simulink model "CMOS_Kernel_Memory_Sync"  (R2023b)
settings: Solver=VariableStepAuto  StartTime=0.0  StopTime=30000000  RelTol=1e-3
values from neighbouring files (symbols this model uses):
  AmountOfPixelsPerScanline = 400    [Kernel_Setup_Script.m]
  AmountOfRamBlocksScanlines = 5    [Kernel_Setup_Script.m]
  AmountOfRamBlocksScanlinesOffset = AmountOfRamBlocksScanlines - 1    (= 4)    [Kernel_Setup_Script.m]
  AmountOfScanlinePixels = 73700    [Kernel_Setup_Script.m]
  AmountOfScanlinePixelsOffset = AmountOfScanlinePixels - 1    (= 73699)    [Kernel_Setup_Script.m]
  AmountOfScanlines = 1100    [Kernel_Setup_Script.m]
  AmountOfScanlinesOffset = AmountOfScanlines - 1    (= 1099)    [Kernel_Setup_Script.m]
  AOPPK_Off = AmountOfPixelsPerScanline - 1    (= 399)    [Kernel_Setup_Script.m]
  AOPPS_Off = AmountOfPixelsPerScanline - 1    (= 399)    [Kernel_Setup_Script.m]
  FramePackOff_0 = FramePackOff_0 - ScanlineFifoCheck    [Kernel_Setup_Script.m]
  FramePackOff_1 = FramePackOff_1 - ScanlineFifoCheck    [Kernel_Setup_Script.m]
  FramePackOff_2 = FramePackOff_2 - ScanlineFifoCheck    [Kernel_Setup_Script.m]
  FramePackOff_3 = FramePackOff_3 - ScanlineFifoCheck    [Kernel_Setup_Script.m]
  FramePackOff_4 = FramePackOff_4 - ScanlineFifoCheck    [Kernel_Setup_Script.m]
  FramePackOff_5 = FramePackOff_5 - ScanlineFifoCheck    [Kernel_Setup_Script.m]
  KernelPackOff_0 = KernelPackOff_0 - KernelBitsPerRow    [Kernel_Setup_Script.m]
  KernelPackOff_1 = KernelPackOff_1 - KernelBitsPerRow    [Kernel_Setup_Script.m]
  KernelPackOff_2 = KernelPackOff_2 - KernelBitsPerRow    [Kernel_Setup_Script.m]
  KernelPackOff_3 = KernelPackOff_3 - KernelBitsPerRow    [Kernel_Setup_Script.m]
  Slice59DownTo48Top = (MsbOffset - (ScanlinePixelBitSizeController*1))    (= 59)    [Kernel_Setup_Script.m]
  Slice71DownTo60Top = (MsbOffset - (ScanlinePixelBitSizeController*0))    (= 71)    [Kernel_Setup_Script.m]
  TotalSectionsForFrames = AmountOfScanlines/AmountOfRamBlocksScanlines    (= 220)    [Kernel_Setup_Script.m]
  UltraRamRows = AmountOfPixelsPerScanline/ScanlineFifoCheck    [Kernel_Setup_Script.m]
  UltraRamRowsCeil = ceil(AmountOfPixelsPerScanline/ScanlineFifoCheck)    [Kernel_Setup_Script.m]
  UltraRamRowsKernel = AmountOfPixelsPerScanline/KernelBitsPerRow    (= 100)    [Kernel_Setup_Script.m]
  UltraRamRowsKernelCeil = ceil(AmountOfPixelsPerScanline/KernelBitsPerRow)    [Kernel_Setup_Script.m]
  UltraRamRowsMemorySectionOffset = UltraRamRowsCeil*AmountOfRamBlocksScanlines    [Kernel_Setup_Script.m]
  UltraRamRowsOffset = UltraRamRowsCeil - 1    [Kernel_Setup_Script.m]
undefined symbols (not defined in the file or in its folder): c, Down, sfvc784, Up, xck26
libraries: hdlBasic x4512, vmcUtilities x1
(part 8 of 39)

== system CMOS_Kernel_Memory_Sync/Memory Handler/Math/Kernel Result 3 ==
  Pixel Bus Input Offset 0 : Inport
  Pixel Bus Input Offset 1 : Inport  Port=2
  Pixel Bus Input Offset 2 : Inport  Port=3
  Pixel Bus Input Offset 3 : Inport  Port=4
  Pixel Bus Input Offset 4 : Inport  Port=5
  Weight Bus Input : Inport  Port=6
  Valid Bus Input : Inport  Port=7
  Hard Reset : Inport  Port=8
  Accumlator Kernel Results : Subsystem
  Accumulator Offset 0 : Subsystem
  Accumulator Offset 1 : Subsystem
  Accumulator Offset 2 : Subsystem
  Accumulator Offset 3 : Subsystem
  Accumulator Offset 4 : Subsystem
  Bus Selector : BusSelector  OutputSignals=signal1,signal2,signal3,signal4,signal5,signal6
  Delay Addition 1 : hdlBasic/Delay  rst=off  en=off  latency=1  reg_retiming=off  XmcBlockStatus=1  maskContainerNames=group1  block_type=delay  block_config=sysgen:Delay_config
  Delay Addition 2 : hdlBasic/Delay  rst=off  en=off  latency=1  reg_retiming=off  XmcBlockStatus=1  maskContainerNames=group1  block_type=delay  block_config=sysgen:Delay_config
  Delay Addition1 : hdlBasic/Delay  rst=off  en=off  latency=3  reg_retiming=off  XmcBlockStatus=1  maskContainerNames=group1  block_type=delay  block_config=sysgen:Delay_config
  Delay Addition{2..4,6..8} (6 alike) : hdlBasic/Delay  rst=off  en=off  latency=1  reg_retiming=off  XmcBlockStatus=1  maskContainerNames=group1  block_type=delay  block_config=sysgen:Delay_config
  Delay Addition5 : hdlBasic/Delay  rst=off  en=off  latency=3  reg_retiming=off  XmcBlockStatus=1  maskContainerNames=group1  block_type=delay  block_config=sysgen:Delay_config
  Multiple and Add Offset 0 : Subsystem
  Multiple and Add Offset 1 : Subsystem
  Multiple and Add Offset 2 : Subsystem
  Multiple and Add Offset 3 : Subsystem
  Multiple and Add Offset 4 : Subsystem
  Pixel Bus Offset {0..4} (5 alike) : BusSelector  OutputSignals=signal1,signal2,signal3,signal4,signal5,signal6,signal7,signal8,signal9,signal10,signal11,signal12
  Valid Selector : BusSelector  OutputSignals=signal1,signal2,signal3,signal4,signal5
  Weight Bus Offset {0..4} (5 alike) : BusSelector  OutputSignals=signal1,signal2,signal3,signal4,signal5,signal6,signal7,signal8,signal9,signal10,signal11,signal12
  Kernel Output : Outport
  Valid Kernel Output : Outport  Port=2
  wires:
  Multiple and Add Offset 4/1(Slice Out) -> Accumulator Offset 4/1(Input Value)
  Accumulator Offset 2/1(Accumulator Output) -> Accumlator Kernel Results/5(Slice Input 2)
  Accumulator Offset 0/2(Accumulator Valid) -> Accumlator Kernel Results/2(Slice Enable 0)
  Accumulator Offset 1/2(Accumulator Valid) -> Accumlator Kernel Results/4(Slice Enable 1)
  Multiple and Add Offset 2/2(Valid Out) -> Accumulator Offset 2/2(Input Valid)
  Accumulator Offset 0/1(Accumulator Output) -> Accumlator Kernel Results/1(Slice Input 0)
  Multiple and Add Offset 0/1(Slice Out) -> Accumulator Offset 0/1(Input Value)
  Multiple and Add Offset 1/1(Slice Out) -> Accumulator Offset 1/1(Input Value)
  Multiple and Add Offset 1/2(Valid Out) -> Accumulator Offset 1/2(Input Valid)
  Accumulator Offset 3/2(Accumulator Valid) -> Accumlator Kernel Results/8(Slice Enable 3)
  Multiple and Add Offset 0/2(Valid Out) -> Accumulator Offset 0/2(Input Valid)
  Multiple and Add Offset 4/2(Valid Out) -> Accumulator Offset 4/2(Input Valid)
  Accumulator Offset 3/1(Accumulator Output) -> Accumlator Kernel Results/7(Slice Input 3)
  Accumulator Offset 2/2(Accumulator Valid) -> Accumlator Kernel Results/6(Slice Enable 2)
  Multiple and Add Offset 3/2(Valid Out) -> Accumulator Offset 3/2(Input Valid)
  Accumulator Offset 4/1(Accumulator Output) -> Accumlator Kernel Results/9(Slice Input 4)
  Multiple and Add Offset 3/1(Slice Out) -> Accumulator Offset 3/1(Input Value)
  Multiple and Add Offset 2/1(Slice Out) -> Accumulator Offset 2/1(Input Value)
  Accumulator Offset 1/1(Accumulator Output) -> Accumlator Kernel Results/3(Slice Input 1)
  Accumulator Offset 4/2(Accumulator Valid) -> Accumlator Kernel Results/10(Slice Enable 4)
  Accumlator Kernel Results/2(Valid Kernel Output) -> Valid Kernel Output/1
  Accumlator Kernel Results/1(Kernel Output) -> Kernel Output/1
  Pixel Bus Input Offset 0/1 -> Pixel Bus Offset 0/1
  Pixel Bus Offset 0/1 -> Multiple and Add Offset 0/1(Pixel 0)  "<signal1>"
  Pixel Bus Offset 0/2 -> Multiple and Add Offset 0/3(Pixel 1)  "<signal2>"
  Pixel Bus Offset 0/3 -> Multiple and Add Offset 0/5(Pixel 2)  "<signal3>"
  Pixel Bus Offset 0/4 -> Multiple and Add Offset 0/7(Pixel 3)  "<signal4>"
  Pixel Bus Offset 0/5 -> Multiple and Add Offset 0/9(Pixel 4)  "<signal5>"
  Pixel Bus Offset 0/6 -> Multiple and Add Offset 0/11(Pixel 5)  "<signal6>"
  Pixel Bus Offset 0/7 -> Multiple and Add Offset 0/13(Pixel 6)  "<signal7>"
  Pixel Bus Offset 0/8 -> Multiple and Add Offset 0/15(Pixel 7)  "<signal8>"
  Pixel Bus Offset 0/9 -> Multiple and Add Offset 0/17(Pixel 8)  "<signal9>"
  Pixel Bus Offset 0/10 -> Multiple and Add Offset 0/19(Pixel 9)  "<signal10>"
  Pixel Bus Offset 0/11 -> Multiple and Add Offset 0/21(Pixel 10)  "<signal11>"
  Pixel Bus Offset 0/12 -> Multiple and Add Offset 0/23(Pixel 11)  "<signal12>"
  Weight Bus Offset 0/1 -> Multiple and Add Offset 0/2(Weight 0)  "<signal1>"
  Weight Bus Offset 0/2 -> Multiple and Add Offset 0/4(Weight 1)  "<signal2>"
  Weight Bus Offset 0/3 -> Multiple and Add Offset 0/6(Weight 2)  "<signal3>"
  Weight Bus Offset 0/4 -> Multiple and Add Offset 0/8(Weight 3)  "<signal4>"
  Weight Bus Offset 0/5 -> Multiple and Add Offset 0/10(Weight 4)  "<signal5>"
  Weight Bus Offset 0/6 -> Multiple and Add Offset 0/12(Weight 5)  "<signal6>"
  Weight Bus Offset 0/7 -> Multiple and Add Offset 0/14(Weight 6)  "<signal7>"
  Weight Bus Offset 0/8 -> Multiple and Add Offset 0/16(Weight 7)  "<signal8>"
  Weight Bus Offset 0/9 -> Multiple and Add Offset 0/18(Weight 8)  "<signal9>"
  Weight Bus Offset 0/10 -> Multiple and Add Offset 0/20(Weight 9)  "<signal10>"
  Weight Bus Offset 0/11 -> Multiple and Add Offset 0/22(Weight 10)  "<signal11>"
  Weight Bus Offset 0/12 -> Multiple and Add Offset 0/24(Weight 11)  "<signal12>"
  Weight Bus Offset 1/5 -> Multiple and Add Offset 1/10(Weight 4)  "<signal5>"
  Pixel Bus Offset 1/7 -> Multiple and Add Offset 1/13(Pixel 6)  "<signal7>"
  Pixel Bus Offset 1/6 -> Multiple and Add Offset 1/11(Pixel 5)  "<signal6>"
  Pixel Bus Offset 1/5 -> Multiple and Add Offset 1/9(Pixel 4)  "<signal5>"
  Pixel Bus Offset 1/3 -> Multiple and Add Offset 1/5(Pixel 2)  "<signal3>"
  Pixel Bus Offset 1/11 -> Multiple and Add Offset 1/21(Pixel 10)  "<signal11>"
  Weight Bus Offset 1/6 -> Multiple and Add Offset 1/12(Weight 5)  "<signal6>"
  Pixel Bus Offset 1/2 -> Multiple and Add Offset 1/3(Pixel 1)  "<signal2>"
  Weight Bus Offset 1/12 -> Multiple and Add Offset 1/24(Weight 11)  "<signal12>"
  Weight Bus Offset 1/1 -> Multiple and Add Offset 1/2(Weight 0)  "<signal1>"
  Pixel Bus Input Offset 1/1 -> Pixel Bus Offset 1/1
  Pixel Bus Offset 1/4 -> Multiple and Add Offset 1/7(Pixel 3)  "<signal4>"
  Weight Bus Offset 1/9 -> Multiple and Add Offset 1/18(Weight 8)  "<signal9>"
  Weight Bus Offset 1/10 -> Multiple and Add Offset 1/20(Weight 9)  "<signal10>"
  Weight Bus Offset 1/11 -> Multiple and Add Offset 1/22(Weight 10)  "<signal11>"
  Weight Bus Offset 1/4 -> Multiple and Add Offset 1/8(Weight 3)  "<signal4>"
  Pixel Bus Offset 1/1 -> Multiple and Add Offset 1/1(Pixel 0)  "<signal1>"
  Weight Bus Offset 1/8 -> Multiple and Add Offset 1/16(Weight 7)  "<signal8>"
  Weight Bus Offset 1/3 -> Multiple and Add Offset 1/6(Weight 2)  "<signal3>"
  Pixel Bus Offset 1/10 -> Multiple and Add Offset 1/19(Pixel 9)  "<signal10>"
  Pixel Bus Offset 1/8 -> Multiple and Add Offset 1/15(Pixel 7)  "<signal8>"
  Pixel Bus Offset 1/12 -> Multiple and Add Offset 1/23(Pixel 11)  "<signal12>"
  Weight Bus Offset 1/7 -> Multiple and Add Offset 1/14(Weight 6)  "<signal7>"
  Weight Bus Offset 1/2 -> Multiple and Add Offset 1/4(Weight 1)  "<signal2>"
  Pixel Bus Offset 1/9 -> Multiple and Add Offset 1/17(Pixel 8)  "<signal9>"
  Weight Bus Offset 2/5 -> Multiple and Add Offset 2/10(Weight 4)  "<signal5>"
  Pixel Bus Offset 2/7 -> Multiple and Add Offset 2/13(Pixel 6)  "<signal7>"
  Pixel Bus Offset 2/6 -> Multiple and Add Offset 2/11(Pixel 5)  "<signal6>"
  Pixel Bus Offset 2/5 -> Multiple and Add Offset 2/9(Pixel 4)  "<signal5>"
  Pixel Bus Offset 2/3 -> Multiple and Add Offset 2/5(Pixel 2)  "<signal3>"
  Pixel Bus Offset 2/11 -> Multiple and Add Offset 2/21(Pixel 10)  "<signal11>"
  Weight Bus Offset 2/6 -> Multiple and Add Offset 2/12(Weight 5)  "<signal6>"
  Pixel Bus Offset 2/2 -> Multiple and Add Offset 2/3(Pixel 1)  "<signal2>"
  Weight Bus Offset 2/12 -> Multiple and Add Offset 2/24(Weight 11)  "<signal12>"
  Weight Bus Offset 2/1 -> Multiple and Add Offset 2/2(Weight 0)  "<signal1>"
  Pixel Bus Input Offset 2/1 -> Pixel Bus Offset 2/1
  Pixel Bus Offset 2/4 -> Multiple and Add Offset 2/7(Pixel 3)  "<signal4>"
  Weight Bus Offset 2/9 -> Multiple and Add Offset 2/18(Weight 8)  "<signal9>"
  Weight Bus Offset 2/10 -> Multiple and Add Offset 2/20(Weight 9)  "<signal10>"
  Weight Bus Offset 2/11 -> Multiple and Add Offset 2/22(Weight 10)  "<signal11>"
  Weight Bus Offset 2/4 -> Multiple and Add Offset 2/8(Weight 3)  "<signal4>"
  Pixel Bus Offset 2/1 -> Multiple and Add Offset 2/1(Pixel 0)  "<signal1>"
  Weight Bus Offset 2/8 -> Multiple and Add Offset 2/16(Weight 7)  "<signal8>"
  Weight Bus Offset 2/3 -> Multiple and Add Offset 2/6(Weight 2)  "<signal3>"
  Pixel Bus Offset 2/10 -> Multiple and Add Offset 2/19(Pixel 9)  "<signal10>"
  Pixel Bus Offset 2/8 -> Multiple and Add Offset 2/15(Pixel 7)  "<signal8>"
  Pixel Bus Offset 2/12 -> Multiple and Add Offset 2/23(Pixel 11)  "<signal12>"
  Weight Bus Offset 2/7 -> Multiple and Add Offset 2/14(Weight 6)  "<signal7>"
  Weight Bus Offset 2/2 -> Multiple and Add Offset 2/4(Weight 1)  "<signal2>"
  Pixel Bus Offset 2/9 -> Multiple and Add Offset 2/17(Pixel 8)  "<signal9>"
  Weight Bus Offset 3/5 -> Multiple and Add Offset 3/10(Weight 4)  "<signal5>"
  Pixel Bus Offset 3/7 -> Multiple and Add Offset 3/13(Pixel 6)  "<signal7>"
  Pixel Bus Offset 3/6 -> Multiple and Add Offset 3/11(Pixel 5)  "<signal6>"
  Pixel Bus Offset 3/5 -> Multiple and Add Offset 3/9(Pixel 4)  "<signal5>"
  Pixel Bus Offset 3/3 -> Multiple and Add Offset 3/5(Pixel 2)  "<signal3>"
  Pixel Bus Offset 3/11 -> Multiple and Add Offset 3/21(Pixel 10)  "<signal11>"
  Weight Bus Offset 3/6 -> Multiple and Add Offset 3/12(Weight 5)  "<signal6>"
  Pixel Bus Offset 3/2 -> Multiple and Add Offset 3/3(Pixel 1)  "<signal2>"
  Weight Bus Offset 3/12 -> Multiple and Add Offset 3/24(Weight 11)  "<signal12>"
  Weight Bus Offset 3/1 -> Multiple and Add Offset 3/2(Weight 0)  "<signal1>"
  Pixel Bus Input Offset 3/1 -> Pixel Bus Offset 3/1
  Pixel Bus Offset 3/4 -> Multiple and Add Offset 3/7(Pixel 3)  "<signal4>"
  Weight Bus Offset 3/9 -> Multiple and Add Offset 3/18(Weight 8)  "<signal9>"
  Weight Bus Offset 3/10 -> Multiple and Add Offset 3/20(Weight 9)  "<signal10>"
  Weight Bus Offset 3/11 -> Multiple and Add Offset 3/22(Weight 10)  "<signal11>"
  Weight Bus Offset 3/4 -> Multiple and Add Offset 3/8(Weight 3)  "<signal4>"
  Pixel Bus Offset 3/1 -> Multiple and Add Offset 3/1(Pixel 0)  "<signal1>"
  Weight Bus Offset 3/8 -> Multiple and Add Offset 3/16(Weight 7)  "<signal8>"
  Weight Bus Offset 3/3 -> Multiple and Add Offset 3/6(Weight 2)  "<signal3>"
  Pixel Bus Offset 3/10 -> Multiple and Add Offset 3/19(Pixel 9)  "<signal10>"
  Pixel Bus Offset 3/8 -> Multiple and Add Offset 3/15(Pixel 7)  "<signal8>"
  Pixel Bus Offset 3/12 -> Multiple and Add Offset 3/23(Pixel 11)  "<signal12>"
  Weight Bus Offset 3/7 -> Multiple and Add Offset 3/14(Weight 6)  "<signal7>"
  Weight Bus Offset 3/2 -> Multiple and Add Offset 3/4(Weight 1)  "<signal2>"
  Pixel Bus Offset 3/9 -> Multiple and Add Offset 3/17(Pixel 8)  "<signal9>"
  Weight Bus Offset 4/5 -> Multiple and Add Offset 4/10(Weight 4)  "<signal5>"
  Pixel Bus Offset 4/7 -> Multiple and Add Offset 4/13(Pixel 6)  "<signal7>"
  Pixel Bus Offset 4/6 -> Multiple and Add Offset 4/11(Pixel 5)  "<signal6>"
  Pixel Bus Offset 4/5 -> Multiple and Add Offset 4/9(Pixel 4)  "<signal5>"
  Pixel Bus Offset 4/3 -> Multiple and Add Offset 4/5(Pixel 2)  "<signal3>"
  Pixel Bus Offset 4/11 -> Multiple and Add Offset 4/21(Pixel 10)  "<signal11>"
  Weight Bus Offset 4/6 -> Multiple and Add Offset 4/12(Weight 5)  "<signal6>"
  Pixel Bus Offset 4/2 -> Multiple and Add Offset 4/3(Pixel 1)  "<signal2>"
  Weight Bus Offset 4/12 -> Multiple and Add Offset 4/24(Weight 11)  "<signal12>"
  Weight Bus Offset 4/1 -> Multiple and Add Offset 4/2(Weight 0)  "<signal1>"
  Pixel Bus Input Offset 4/1 -> Pixel Bus Offset 4/1
  Pixel Bus Offset 4/4 -> Multiple and Add Offset 4/7(Pixel 3)  "<signal4>"
  Weight Bus Offset 4/9 -> Multiple and Add Offset 4/18(Weight 8)  "<signal9>"
  Weight Bus Offset 4/10 -> Multiple and Add Offset 4/20(Weight 9)  "<signal10>"
  Weight Bus Offset 4/11 -> Multiple and Add Offset 4/22(Weight 10)  "<signal11>"
  Weight Bus Offset 4/4 -> Multiple and Add Offset 4/8(Weight 3)  "<signal4>"
  Pixel Bus Offset 4/1 -> Multiple and Add Offset 4/1(Pixel 0)  "<signal1>"
  Weight Bus Offset 4/8 -> Multiple and Add Offset 4/16(Weight 7)  "<signal8>"
  Weight Bus Offset 4/3 -> Multiple and Add Offset 4/6(Weight 2)  "<signal3>"
  Pixel Bus Offset 4/10 -> Multiple and Add Offset 4/19(Pixel 9)  "<signal10>"
  Pixel Bus Offset 4/8 -> Multiple and Add Offset 4/15(Pixel 7)  "<signal8>"
  Pixel Bus Offset 4/12 -> Multiple and Add Offset 4/23(Pixel 11)  "<signal12>"
  Weight Bus Offset 4/7 -> Multiple and Add Offset 4/14(Weight 6)  "<signal7>"
  Weight Bus Offset 4/2 -> Multiple and Add Offset 4/4(Weight 1)  "<signal2>"
  Pixel Bus Offset 4/9 -> Multiple and Add Offset 4/17(Pixel 8)  "<signal9>"
  Valid Bus Input/1 -> Valid Selector/1
  Valid Selector/1 -> Multiple and Add Offset 0/25(Valid Data)  "<signal1>"
  Valid Selector/2 -> Multiple and Add Offset 1/25(Valid Data)  "<signal2>"
  Valid Selector/3 -> Multiple and Add Offset 2/25(Valid Data)  "<signal3>"
  Valid Selector/4 -> Multiple and Add Offset 3/25(Valid Data)  "<signal4>"
  Valid Selector/5 -> Multiple and Add Offset 4/25(Valid Data)  "<signal5>"
  Weight Bus Input/1 -> Bus Selector/1
  Bus Selector/5 -> Weight Bus Offset 4/1  "<signal5>"
  Bus Selector/4 -> Weight Bus Offset 3/1  "<signal4>"
  Bus Selector/3 -> Weight Bus Offset 2/1  "<signal3>"
  Bus Selector/2 -> Weight Bus Offset 1/1  "<signal2>"
  Bus Selector/1 -> Weight Bus Offset 0/1  "<signal1>"
  Delay Addition4/1 -> Accumulator Offset 4/3(Last Row), Accumulator Offset 3/3(Last Row), Accumulator Offset 2/3(Last Row), Accumulator Offset 1/3(Last Row), Accumulator Offset 0/3(Last Row)
  Delay Addition 2/1 -> Delay Addition2/1
  Delay Addition1/1 -> Delay Addition 2/1
  Delay Addition2/1 -> Delay Addition3/1
  Delay Addition3/1 -> Delay Addition4/1
  Bus Selector/6 -> Delay Addition1/1  "<signal6>"
  Delay Addition7/1 -> Delay Addition8/1
  Delay Addition 1/1 -> Delay Addition6/1
  Delay Addition5/1 -> Delay Addition 1/1
  Delay Addition6/1 -> Delay Addition7/1
  Delay Addition8/1 -> Accumlator Kernel Results/11(Reset Collector), Accumulator Offset 0/4(Hard Reset), Accumulator Offset 1/4(Hard Reset), Accumulator Offset 2/4(Hard Reset), Accumulator Offset 3/4(Hard Reset), Accumulator Offset 4/4(Hard Reset)
  Hard Reset/1 -> Delay Addition5/1

== system CMOS_Kernel_Memory_Sync/Memory Handler/Math/Kernel Result 4 ==
  Pixel Bus Input Offset 0 : Inport
  Pixel Bus Input Offset 1 : Inport  Port=2
  Pixel Bus Input Offset 2 : Inport  Port=3
  Pixel Bus Input Offset 3 : Inport  Port=4
  Pixel Bus Input Offset 4 : Inport  Port=5
  Weight Bus Input : Inport  Port=6
  Valid Bus Input : Inport  Port=7
  Hard Reset : Inport  Port=8
  Accumlator Kernel Results : Subsystem
  Accumulator Offset 0 : Subsystem
  Accumulator Offset 1 : Subsystem
  Accumulator Offset 2 : Subsystem
  Accumulator Offset 3 : Subsystem
  Accumulator Offset 4 : Subsystem
  Bus Selector : BusSelector  OutputSignals=signal1,signal2,signal3,signal4,signal5,signal6
  Delay Addition 1 : hdlBasic/Delay  rst=off  en=off  latency=1  reg_retiming=off  XmcBlockStatus=1  maskContainerNames=group1  block_type=delay  block_config=sysgen:Delay_config
  Delay Addition 2 : hdlBasic/Delay  rst=off  en=off  latency=1  reg_retiming=off  XmcBlockStatus=1  maskContainerNames=group1  block_type=delay  block_config=sysgen:Delay_config
  Delay Addition1 : hdlBasic/Delay  rst=off  en=off  latency=3  reg_retiming=off  XmcBlockStatus=1  maskContainerNames=group1  block_type=delay  block_config=sysgen:Delay_config
  Delay Addition{2..4,6..8} (6 alike) : hdlBasic/Delay  rst=off  en=off  latency=1  reg_retiming=off  XmcBlockStatus=1  maskContainerNames=group1  block_type=delay  block_config=sysgen:Delay_config
  Delay Addition5 : hdlBasic/Delay  rst=off  en=off  latency=3  reg_retiming=off  XmcBlockStatus=1  maskContainerNames=group1  block_type=delay  block_config=sysgen:Delay_config
  Multiple and Add Offset 0 : Subsystem
  Multiple and Add Offset 1 : Subsystem
  Multiple and Add Offset 2 : Subsystem
  Multiple and Add Offset 3 : Subsystem
  Multiple and Add Offset 4 : Subsystem
  Pixel Bus Offset {0..4} (5 alike) : BusSelector  OutputSignals=signal1,signal2,signal3,signal4,signal5,signal6,signal7,signal8,signal9,signal10,signal11,signal12
  Valid Selector : BusSelector  OutputSignals=signal1,signal2,signal3,signal4,signal5
  Weight Bus Offset {0..4} (5 alike) : BusSelector  OutputSignals=signal1,signal2,signal3,signal4,signal5,signal6,signal7,signal8,signal9,signal10,signal11,signal12
  Kernel Output : Outport
  Valid Kernel Output : Outport  Port=2
  wires:
  Multiple and Add Offset 4/1(Slice Out) -> Accumulator Offset 4/1(Input Value)
  Accumulator Offset 2/1(Accumulator Output) -> Accumlator Kernel Results/5(Slice Input 2)
  Accumulator Offset 0/2(Accumulator Valid) -> Accumlator Kernel Results/2(Slice Enable 0)
  Accumulator Offset 1/2(Accumulator Valid) -> Accumlator Kernel Results/4(Slice Enable 1)
  Multiple and Add Offset 2/2(Valid Out) -> Accumulator Offset 2/2(Input Valid)
  Accumulator Offset 0/1(Accumulator Output) -> Accumlator Kernel Results/1(Slice Input 0)
  Multiple and Add Offset 0/1(Slice Out) -> Accumulator Offset 0/1(Input Value)
  Multiple and Add Offset 1/1(Slice Out) -> Accumulator Offset 1/1(Input Value)
  Multiple and Add Offset 1/2(Valid Out) -> Accumulator Offset 1/2(Input Valid)
  Accumulator Offset 3/2(Accumulator Valid) -> Accumlator Kernel Results/8(Slice Enable 3)
  Multiple and Add Offset 0/2(Valid Out) -> Accumulator Offset 0/2(Input Valid)
  Multiple and Add Offset 4/2(Valid Out) -> Accumulator Offset 4/2(Input Valid)
  Accumulator Offset 3/1(Accumulator Output) -> Accumlator Kernel Results/7(Slice Input 3)
  Accumulator Offset 2/2(Accumulator Valid) -> Accumlator Kernel Results/6(Slice Enable 2)
  Multiple and Add Offset 3/2(Valid Out) -> Accumulator Offset 3/2(Input Valid)
  Accumulator Offset 4/1(Accumulator Output) -> Accumlator Kernel Results/9(Slice Input 4)
  Multiple and Add Offset 3/1(Slice Out) -> Accumulator Offset 3/1(Input Value)
  Multiple and Add Offset 2/1(Slice Out) -> Accumulator Offset 2/1(Input Value)
  Accumulator Offset 1/1(Accumulator Output) -> Accumlator Kernel Results/3(Slice Input 1)
  Accumulator Offset 4/2(Accumulator Valid) -> Accumlator Kernel Results/10(Slice Enable 4)
  Accumlator Kernel Results/2(Valid Kernel Output) -> Valid Kernel Output/1
  Accumlator Kernel Results/1(Kernel Output) -> Kernel Output/1
  Pixel Bus Input Offset 0/1 -> Pixel Bus Offset 0/1
  Pixel Bus Offset 0/1 -> Multiple and Add Offset 0/1(Pixel 0)  "<signal1>"
  Pixel Bus Offset 0/2 -> Multiple and Add Offset 0/3(Pixel 1)  "<signal2>"
  Pixel Bus Offset 0/3 -> Multiple and Add Offset 0/5(Pixel 2)  "<signal3>"
  Pixel Bus Offset 0/4 -> Multiple and Add Offset 0/7(Pixel 3)  "<signal4>"
  Pixel Bus Offset 0/5 -> Multiple and Add Offset 0/9(Pixel 4)  "<signal5>"
  Pixel Bus Offset 0/6 -> Multiple and Add Offset 0/11(Pixel 5)  "<signal6>"
  Pixel Bus Offset 0/7 -> Multiple and Add Offset 0/13(Pixel 6)  "<signal7>"
  Pixel Bus Offset 0/8 -> Multiple and Add Offset 0/15(Pixel 7)  "<signal8>"
  Pixel Bus Offset 0/9 -> Multiple and Add Offset 0/17(Pixel 8)  "<signal9>"
  Pixel Bus Offset 0/10 -> Multiple and Add Offset 0/19(Pixel 9)  "<signal10>"
  Pixel Bus Offset 0/11 -> Multiple and Add Offset 0/21(Pixel 10)  "<signal11>"
  Pixel Bus Offset 0/12 -> Multiple and Add Offset 0/23(Pixel 11)  "<signal12>"
  Weight Bus Offset 0/1 -> Multiple and Add Offset 0/2(Weight 0)  "<signal1>"
  Weight Bus Offset 0/2 -> Multiple and Add Offset 0/4(Weight 1)  "<signal2>"
  Weight Bus Offset 0/3 -> Multiple and Add Offset 0/6(Weight 2)  "<signal3>"
  Weight Bus Offset 0/4 -> Multiple and Add Offset 0/8(Weight 3)  "<signal4>"
  Weight Bus Offset 0/5 -> Multiple and Add Offset 0/10(Weight 4)  "<signal5>"
  Weight Bus Offset 0/6 -> Multiple and Add Offset 0/12(Weight 5)  "<signal6>"
  Weight Bus Offset 0/7 -> Multiple and Add Offset 0/14(Weight 6)  "<signal7>"
  Weight Bus Offset 0/8 -> Multiple and Add Offset 0/16(Weight 7)  "<signal8>"
  Weight Bus Offset 0/9 -> Multiple and Add Offset 0/18(Weight 8)  "<signal9>"
  Weight Bus Offset 0/10 -> Multiple and Add Offset 0/20(Weight 9)  "<signal10>"
  Weight Bus Offset 0/11 -> Multiple and Add Offset 0/22(Weight 10)  "<signal11>"
  Weight Bus Offset 0/12 -> Multiple and Add Offset 0/24(Weight 11)  "<signal12>"
  Weight Bus Offset 1/5 -> Multiple and Add Offset 1/10(Weight 4)  "<signal5>"
  Pixel Bus Offset 1/7 -> Multiple and Add Offset 1/13(Pixel 6)  "<signal7>"
  Pixel Bus Offset 1/6 -> Multiple and Add Offset 1/11(Pixel 5)  "<signal6>"
  Pixel Bus Offset 1/5 -> Multiple and Add Offset 1/9(Pixel 4)  "<signal5>"
  Pixel Bus Offset 1/3 -> Multiple and Add Offset 1/5(Pixel 2)  "<signal3>"
  Pixel Bus Offset 1/11 -> Multiple and Add Offset 1/21(Pixel 10)  "<signal11>"
  Weight Bus Offset 1/6 -> Multiple and Add Offset 1/12(Weight 5)  "<signal6>"
  Pixel Bus Offset 1/2 -> Multiple and Add Offset 1/3(Pixel 1)  "<signal2>"
  Weight Bus Offset 1/12 -> Multiple and Add Offset 1/24(Weight 11)  "<signal12>"
  Weight Bus Offset 1/1 -> Multiple and Add Offset 1/2(Weight 0)  "<signal1>"
  Pixel Bus Input Offset 1/1 -> Pixel Bus Offset 1/1
  Pixel Bus Offset 1/4 -> Multiple and Add Offset 1/7(Pixel 3)  "<signal4>"
  Weight Bus Offset 1/9 -> Multiple and Add Offset 1/18(Weight 8)  "<signal9>"
  Weight Bus Offset 1/10 -> Multiple and Add Offset 1/20(Weight 9)  "<signal10>"
  Weight Bus Offset 1/11 -> Multiple and Add Offset 1/22(Weight 10)  "<signal11>"
  Weight Bus Offset 1/4 -> Multiple and Add Offset 1/8(Weight 3)  "<signal4>"
  Pixel Bus Offset 1/1 -> Multiple and Add Offset 1/1(Pixel 0)  "<signal1>"
  Weight Bus Offset 1/8 -> Multiple and Add Offset 1/16(Weight 7)  "<signal8>"
  Weight Bus Offset 1/3 -> Multiple and Add Offset 1/6(Weight 2)  "<signal3>"
  Pixel Bus Offset 1/10 -> Multiple and Add Offset 1/19(Pixel 9)  "<signal10>"
  Pixel Bus Offset 1/8 -> Multiple and Add Offset 1/15(Pixel 7)  "<signal8>"
  Pixel Bus Offset 1/12 -> Multiple and Add Offset 1/23(Pixel 11)  "<signal12>"
  Weight Bus Offset 1/7 -> Multiple and Add Offset 1/14(Weight 6)  "<signal7>"
  Weight Bus Offset 1/2 -> Multiple and Add Offset 1/4(Weight 1)  "<signal2>"
  Pixel Bus Offset 1/9 -> Multiple and Add Offset 1/17(Pixel 8)  "<signal9>"
  Weight Bus Offset 2/5 -> Multiple and Add Offset 2/10(Weight 4)  "<signal5>"
  Pixel Bus Offset 2/7 -> Multiple and Add Offset 2/13(Pixel 6)  "<signal7>"
  Pixel Bus Offset 2/6 -> Multiple and Add Offset 2/11(Pixel 5)  "<signal6>"
  Pixel Bus Offset 2/5 -> Multiple and Add Offset 2/9(Pixel 4)  "<signal5>"
  Pixel Bus Offset 2/3 -> Multiple and Add Offset 2/5(Pixel 2)  "<signal3>"
  Pixel Bus Offset 2/11 -> Multiple and Add Offset 2/21(Pixel 10)  "<signal11>"
  Weight Bus Offset 2/6 -> Multiple and Add Offset 2/12(Weight 5)  "<signal6>"
  Pixel Bus Offset 2/2 -> Multiple and Add Offset 2/3(Pixel 1)  "<signal2>"
  Weight Bus Offset 2/12 -> Multiple and Add Offset 2/24(Weight 11)  "<signal12>"
  Weight Bus Offset 2/1 -> Multiple and Add Offset 2/2(Weight 0)  "<signal1>"
  Pixel Bus Input Offset 2/1 -> Pixel Bus Offset 2/1
  Pixel Bus Offset 2/4 -> Multiple and Add Offset 2/7(Pixel 3)  "<signal4>"
  Weight Bus Offset 2/9 -> Multiple and Add Offset 2/18(Weight 8)  "<signal9>"
  Weight Bus Offset 2/10 -> Multiple and Add Offset 2/20(Weight 9)  "<signal10>"
  Weight Bus Offset 2/11 -> Multiple and Add Offset 2/22(Weight 10)  "<signal11>"
  Weight Bus Offset 2/4 -> Multiple and Add Offset 2/8(Weight 3)  "<signal4>"
  Pixel Bus Offset 2/1 -> Multiple and Add Offset 2/1(Pixel 0)  "<signal1>"
  Weight Bus Offset 2/8 -> Multiple and Add Offset 2/16(Weight 7)  "<signal8>"
  Weight Bus Offset 2/3 -> Multiple and Add Offset 2/6(Weight 2)  "<signal3>"
  Pixel Bus Offset 2/10 -> Multiple and Add Offset 2/19(Pixel 9)  "<signal10>"
  Pixel Bus Offset 2/8 -> Multiple and Add Offset 2/15(Pixel 7)  "<signal8>"
  Pixel Bus Offset 2/12 -> Multiple and Add Offset 2/23(Pixel 11)  "<signal12>"
  Weight Bus Offset 2/7 -> Multiple and Add Offset 2/14(Weight 6)  "<signal7>"
  Weight Bus Offset 2/2 -> Multiple and Add Offset 2/4(Weight 1)  "<signal2>"
  Pixel Bus Offset 2/9 -> Multiple and Add Offset 2/17(Pixel 8)  "<signal9>"
  Weight Bus Offset 3/5 -> Multiple and Add Offset 3/10(Weight 4)  "<signal5>"
  Pixel Bus Offset 3/7 -> Multiple and Add Offset 3/13(Pixel 6)  "<signal7>"
  Pixel Bus Offset 3/6 -> Multiple and Add Offset 3/11(Pixel 5)  "<signal6>"
  Pixel Bus Offset 3/5 -> Multiple and Add Offset 3/9(Pixel 4)  "<signal5>"
  Pixel Bus Offset 3/3 -> Multiple and Add Offset 3/5(Pixel 2)  "<signal3>"
  Pixel Bus Offset 3/11 -> Multiple and Add Offset 3/21(Pixel 10)  "<signal11>"
  Weight Bus Offset 3/6 -> Multiple and Add Offset 3/12(Weight 5)  "<signal6>"
  Pixel Bus Offset 3/2 -> Multiple and Add Offset 3/3(Pixel 1)  "<signal2>"
  Weight Bus Offset 3/12 -> Multiple and Add Offset 3/24(Weight 11)  "<signal12>"
  Weight Bus Offset 3/1 -> Multiple and Add Offset 3/2(Weight 0)  "<signal1>"
  Pixel Bus Input Offset 3/1 -> Pixel Bus Offset 3/1
  Pixel Bus Offset 3/4 -> Multiple and Add Offset 3/7(Pixel 3)  "<signal4>"
  Weight Bus Offset 3/9 -> Multiple and Add Offset 3/18(Weight 8)  "<signal9>"
  Weight Bus Offset 3/10 -> Multiple and Add Offset 3/20(Weight 9)  "<signal10>"
  Weight Bus Offset 3/11 -> Multiple and Add Offset 3/22(Weight 10)  "<signal11>"
  Weight Bus Offset 3/4 -> Multiple and Add Offset 3/8(Weight 3)  "<signal4>"
  Pixel Bus Offset 3/1 -> Multiple and Add Offset 3/1(Pixel 0)  "<signal1>"
  Weight Bus Offset 3/8 -> Multiple and Add Offset 3/16(Weight 7)  "<signal8>"
  Weight Bus Offset 3/3 -> Multiple and Add Offset 3/6(Weight 2)  "<signal3>"
  Pixel Bus Offset 3/10 -> Multiple and Add Offset 3/19(Pixel 9)  "<signal10>"
  Pixel Bus Offset 3/8 -> Multiple and Add Offset 3/15(Pixel 7)  "<signal8>"
  Pixel Bus Offset 3/12 -> Multiple and Add Offset 3/23(Pixel 11)  "<signal12>"
  Weight Bus Offset 3/7 -> Multiple and Add Offset 3/14(Weight 6)  "<signal7>"
  Weight Bus Offset 3/2 -> Multiple and Add Offset 3/4(Weight 1)  "<signal2>"
  Pixel Bus Offset 3/9 -> Multiple and Add Offset 3/17(Pixel 8)  "<signal9>"
  Weight Bus Offset 4/5 -> Multiple and Add Offset 4/10(Weight 4)  "<signal5>"
  Pixel Bus Offset 4/7 -> Multiple and Add Offset 4/13(Pixel 6)  "<signal7>"
  Pixel Bus Offset 4/6 -> Multiple and Add Offset 4/11(Pixel 5)  "<signal6>"
  Pixel Bus Offset 4/5 -> Multiple and Add Offset 4/9(Pixel 4)  "<signal5>"
  Pixel Bus Offset 4/3 -> Multiple and Add Offset 4/5(Pixel 2)  "<signal3>"
  Pixel Bus Offset 4/11 -> Multiple and Add Offset 4/21(Pixel 10)  "<signal11>"
  Weight Bus Offset 4/6 -> Multiple and Add Offset 4/12(Weight 5)  "<signal6>"
  Pixel Bus Offset 4/2 -> Multiple and Add Offset 4/3(Pixel 1)  "<signal2>"
  Weight Bus Offset 4/12 -> Multiple and Add Offset 4/24(Weight 11)  "<signal12>"
  Weight Bus Offset 4/1 -> Multiple and Add Offset 4/2(Weight 0)  "<signal1>"
  Pixel Bus Input Offset 4/1 -> Pixel Bus Offset 4/1
  Pixel Bus Offset 4/4 -> Multiple and Add Offset 4/7(Pixel 3)  "<signal4>"
  Weight Bus Offset 4/9 -> Multiple and Add Offset 4/18(Weight 8)  "<signal9>"
  Weight Bus Offset 4/10 -> Multiple and Add Offset 4/20(Weight 9)  "<signal10>"
  Weight Bus Offset 4/11 -> Multiple and Add Offset 4/22(Weight 10)  "<signal11>"
  Weight Bus Offset 4/4 -> Multiple and Add Offset 4/8(Weight 3)  "<signal4>"
  Pixel Bus Offset 4/1 -> Multiple and Add Offset 4/1(Pixel 0)  "<signal1>"
  Weight Bus Offset 4/8 -> Multiple and Add Offset 4/16(Weight 7)  "<signal8>"
  Weight Bus Offset 4/3 -> Multiple and Add Offset 4/6(Weight 2)  "<signal3>"
  Pixel Bus Offset 4/10 -> Multiple and Add Offset 4/19(Pixel 9)  "<signal10>"
  Pixel Bus Offset 4/8 -> Multiple and Add Offset 4/15(Pixel 7)  "<signal8>"
  Pixel Bus Offset 4/12 -> Multiple and Add Offset 4/23(Pixel 11)  "<signal12>"
  Weight Bus Offset 4/7 -> Multiple and Add Offset 4/14(Weight 6)  "<signal7>"
  Weight Bus Offset 4/2 -> Multiple and Add Offset 4/4(Weight 1)  "<signal2>"
  Pixel Bus Offset 4/9 -> Multiple and Add Offset 4/17(Pixel 8)  "<signal9>"
  Valid Bus Input/1 -> Valid Selector/1
  Valid Selector/1 -> Multiple and Add Offset 0/25(Valid Data)  "<signal1>"
  Valid Selector/2 -> Multiple and Add Offset 1/25(Valid Data)  "<signal2>"
  Valid Selector/3 -> Multiple and Add Offset 2/25(Valid Data)  "<signal3>"
  Valid Selector/4 -> Multiple and Add Offset 3/25(Valid Data)  "<signal4>"
  Valid Selector/5 -> Multiple and Add Offset 4/25(Valid Data)  "<signal5>"
  Weight Bus Input/1 -> Bus Selector/1
  Bus Selector/5 -> Weight Bus Offset 4/1  "<signal5>"
  Bus Selector/4 -> Weight Bus Offset 3/1  "<signal4>"
  Bus Selector/3 -> Weight Bus Offset 2/1  "<signal3>"
  Bus Selector/2 -> Weight Bus Offset 1/1  "<signal2>"
  Bus Selector/1 -> Weight Bus Offset 0/1  "<signal1>"
  Delay Addition4/1 -> Accumulator Offset 4/3(Last Row), Accumulator Offset 3/3(Last Row), Accumulator Offset 2/3(Last Row), Accumulator Offset 1/3(Last Row), Accumulator Offset 0/3(Last Row)
  Delay Addition 2/1 -> Delay Addition2/1
  Delay Addition1/1 -> Delay Addition 2/1
  Delay Addition2/1 -> Delay Addition3/1
  Delay Addition3/1 -> Delay Addition4/1
  Bus Selector/6 -> Delay Addition1/1  "<signal6>"
  Delay Addition7/1 -> Delay Addition8/1
  Delay Addition 1/1 -> Delay Addition6/1
  Delay Addition5/1 -> Delay Addition 1/1
  Delay Addition6/1 -> Delay Addition7/1
  Delay Addition8/1 -> Accumlator Kernel Results/11(Reset Collector), Accumulator Offset 0/4(Hard Reset), Accumulator Offset 1/4(Hard Reset), Accumulator Offset 2/4(Hard Reset), Accumulator Offset 3/4(Hard Reset), Accumulator Offset 4/4(Hard Reset)
  Hard Reset/1 -> Delay Addition5/1

== system CMOS_Kernel_Memory_Sync/Memory Handler/Math/Kernel Result 5 ==
  Pixel Bus Input Offset 0 : Inport
  Pixel Bus Input Offset 1 : Inport  Port=2
  Pixel Bus Input Offset 2 : Inport  Port=3
  Pixel Bus Input Offset 3 : Inport  Port=4
  Pixel Bus Input Offset 4 : Inport  Port=5
  Weight Bus Input : Inport  Port=6
  Valid Bus Input : Inport  Port=7
  Hard Reset : Inport  Port=8
  Accumlator Kernel Results : Subsystem
  Accumulator Offset 0 : Subsystem
  Accumulator Offset 1 : Subsystem
  Accumulator Offset 2 : Subsystem
  Accumulator Offset 3 : Subsystem
  Accumulator Offset 4 : Subsystem
  Bus Selector : BusSelector  OutputSignals=signal1,signal2,signal3,signal4,signal5,signal6
  Delay Addition 1 : hdlBasic/Delay  rst=off  en=off  latency=1  reg_retiming=off  XmcBlockStatus=1  maskContainerNames=group1  block_type=delay  block_config=sysgen:Delay_config
  Delay Addition 2 : hdlBasic/Delay  rst=off  en=off  latency=1  reg_retiming=off  XmcBlockStatus=1  maskContainerNames=group1  block_type=delay  block_config=sysgen:Delay_config
  Delay Addition1 : hdlBasic/Delay  rst=off  en=off  latency=3  reg_retiming=off  XmcBlockStatus=1  maskContainerNames=group1  block_type=delay  block_config=sysgen:Delay_config
  Delay Addition{2..4,6..8} (6 alike) : hdlBasic/Delay  rst=off  en=off  latency=1  reg_retiming=off  XmcBlockStatus=1  maskContainerNames=group1  block_type=delay  block_config=sysgen:Delay_config
  Delay Addition5 : hdlBasic/Delay  rst=off  en=off  latency=3  reg_retiming=off  XmcBlockStatus=1  maskContainerNames=group1  block_type=delay  block_config=sysgen:Delay_config
  Multiple and Add Offset 0 : Subsystem
  Multiple and Add Offset 1 : Subsystem
  Multiple and Add Offset 2 : Subsystem
  Multiple and Add Offset 3 : Subsystem
  Multiple and Add Offset 4 : Subsystem
  Pixel Bus Offset {0..4} (5 alike) : BusSelector  OutputSignals=signal1,signal2,signal3,signal4,signal5,signal6,signal7,signal8,signal9,signal10,signal11,signal12
  Valid Selector : BusSelector  OutputSignals=signal1,signal2,signal3,signal4,signal5
  Weight Bus Offset {0..4} (5 alike) : BusSelector  OutputSignals=signal1,signal2,signal3,signal4,signal5,signal6,signal7,signal8,signal9,signal10,signal11,signal12
  Kernel Output : Outport
  Valid Kernel Output : Outport  Port=2
  wires:
  Multiple and Add Offset 4/1(Slice Out) -> Accumulator Offset 4/1(Input Value)
  Accumulator Offset 2/1(Accumulator Output) -> Accumlator Kernel Results/5(Slice Input 2)
  Accumulator Offset 0/2(Accumulator Valid) -> Accumlator Kernel Results/2(Slice Enable 0)
  Accumulator Offset 1/2(Accumulator Valid) -> Accumlator Kernel Results/4(Slice Enable 1)
  Multiple and Add Offset 2/2(Valid Out) -> Accumulator Offset 2/2(Input Valid)
  Accumulator Offset 0/1(Accumulator Output) -> Accumlator Kernel Results/1(Slice Input 0)
  Multiple and Add Offset 0/1(Slice Out) -> Accumulator Offset 0/1(Input Value)
  Multiple and Add Offset 1/1(Slice Out) -> Accumulator Offset 1/1(Input Value)
  Multiple and Add Offset 1/2(Valid Out) -> Accumulator Offset 1/2(Input Valid)
  Accumulator Offset 3/2(Accumulator Valid) -> Accumlator Kernel Results/8(Slice Enable 3)
  Multiple and Add Offset 0/2(Valid Out) -> Accumulator Offset 0/2(Input Valid)
  Multiple and Add Offset 4/2(Valid Out) -> Accumulator Offset 4/2(Input Valid)
  Accumulator Offset 3/1(Accumulator Output) -> Accumlator Kernel Results/7(Slice Input 3)
  Accumulator Offset 2/2(Accumulator Valid) -> Accumlator Kernel Results/6(Slice Enable 2)
  Multiple and Add Offset 3/2(Valid Out) -> Accumulator Offset 3/2(Input Valid)
  Accumulator Offset 4/1(Accumulator Output) -> Accumlator Kernel Results/9(Slice Input 4)
  Multiple and Add Offset 3/1(Slice Out) -> Accumulator Offset 3/1(Input Value)
  Multiple and Add Offset 2/1(Slice Out) -> Accumulator Offset 2/1(Input Value)
  Accumulator Offset 1/1(Accumulator Output) -> Accumlator Kernel Results/3(Slice Input 1)
  Accumulator Offset 4/2(Accumulator Valid) -> Accumlator Kernel Results/10(Slice Enable 4)
  Accumlator Kernel Results/2(Valid Kernel Output) -> Valid Kernel Output/1
  Accumlator Kernel Results/1(Kernel Output) -> Kernel Output/1
  Pixel Bus Input Offset 0/1 -> Pixel Bus Offset 0/1
  Pixel Bus Offset 0/1 -> Multiple and Add Offset 0/1(Pixel 0)  "<signal1>"
  Pixel Bus Offset 0/2 -> Multiple and Add Offset 0/3(Pixel 1)  "<signal2>"
  Pixel Bus Offset 0/3 -> Multiple and Add Offset 0/5(Pixel 2)  "<signal3>"
  Pixel Bus Offset 0/4 -> Multiple and Add Offset 0/7(Pixel 3)  "<signal4>"
  Pixel Bus Offset 0/5 -> Multiple and Add Offset 0/9(Pixel 4)  "<signal5>"
  Pixel Bus Offset 0/6 -> Multiple and Add Offset 0/11(Pixel 5)  "<signal6>"
  Pixel Bus Offset 0/7 -> Multiple and Add Offset 0/13(Pixel 6)  "<signal7>"
  Pixel Bus Offset 0/8 -> Multiple and Add Offset 0/15(Pixel 7)  "<signal8>"
  Pixel Bus Offset 0/9 -> Multiple and Add Offset 0/17(Pixel 8)  "<signal9>"
  Pixel Bus Offset 0/10 -> Multiple and Add Offset 0/19(Pixel 9)  "<signal10>"
  Pixel Bus Offset 0/11 -> Multiple and Add Offset 0/21(Pixel 10)  "<signal11>"
  Pixel Bus Offset 0/12 -> Multiple and Add Offset 0/23(Pixel 11)  "<signal12>"
  Weight Bus Offset 0/1 -> Multiple and Add Offset 0/2(Weight 0)  "<signal1>"
  Weight Bus Offset 0/2 -> Multiple and Add Offset 0/4(Weight 1)  "<signal2>"
  Weight Bus Offset 0/3 -> Multiple and Add Offset 0/6(Weight 2)  "<signal3>"
  Weight Bus Offset 0/4 -> Multiple and Add Offset 0/8(Weight 3)  "<signal4>"
  Weight Bus Offset 0/5 -> Multiple and Add Offset 0/10(Weight 4)  "<signal5>"
  Weight Bus Offset 0/6 -> Multiple and Add Offset 0/12(Weight 5)  "<signal6>"
  Weight Bus Offset 0/7 -> Multiple and Add Offset 0/14(Weight 6)  "<signal7>"
  Weight Bus Offset 0/8 -> Multiple and Add Offset 0/16(Weight 7)  "<signal8>"
  Weight Bus Offset 0/9 -> Multiple and Add Offset 0/18(Weight 8)  "<signal9>"
  Weight Bus Offset 0/10 -> Multiple and Add Offset 0/20(Weight 9)  "<signal10>"
  Weight Bus Offset 0/11 -> Multiple and Add Offset 0/22(Weight 10)  "<signal11>"
  Weight Bus Offset 0/12 -> Multiple and Add Offset 0/24(Weight 11)  "<signal12>"
  Weight Bus Offset 1/5 -> Multiple and Add Offset 1/10(Weight 4)  "<signal5>"
  Pixel Bus Offset 1/7 -> Multiple and Add Offset 1/13(Pixel 6)  "<signal7>"
  Pixel Bus Offset 1/6 -> Multiple and Add Offset 1/11(Pixel 5)  "<signal6>"
  Pixel Bus Offset 1/5 -> Multiple and Add Offset 1/9(Pixel 4)  "<signal5>"
  Pixel Bus Offset 1/3 -> Multiple and Add Offset 1/5(Pixel 2)  "<signal3>"
  Pixel Bus Offset 1/11 -> Multiple and Add Offset 1/21(Pixel 10)  "<signal11>"
  Weight Bus Offset 1/6 -> Multiple and Add Offset 1/12(Weight 5)  "<signal6>"
  Pixel Bus Offset 1/2 -> Multiple and Add Offset 1/3(Pixel 1)  "<signal2>"
  Weight Bus Offset 1/12 -> Multiple and Add Offset 1/24(Weight 11)  "<signal12>"
  Weight Bus Offset 1/1 -> Multiple and Add Offset 1/2(Weight 0)  "<signal1>"
  Pixel Bus Input Offset 1/1 -> Pixel Bus Offset 1/1
  Pixel Bus Offset 1/4 -> Multiple and Add Offset 1/7(Pixel 3)  "<signal4>"
  Weight Bus Offset 1/9 -> Multiple and Add Offset 1/18(Weight 8)  "<signal9>"
  Weight Bus Offset 1/10 -> Multiple and Add Offset 1/20(Weight 9)  "<signal10>"
  Weight Bus Offset 1/11 -> Multiple and Add Offset 1/22(Weight 10)  "<signal11>"
  Weight Bus Offset 1/4 -> Multiple and Add Offset 1/8(Weight 3)  "<signal4>"
  Pixel Bus Offset 1/1 -> Multiple and Add Offset 1/1(Pixel 0)  "<signal1>"
  Weight Bus Offset 1/8 -> Multiple and Add Offset 1/16(Weight 7)  "<signal8>"
  Weight Bus Offset 1/3 -> Multiple and Add Offset 1/6(Weight 2)  "<signal3>"
  Pixel Bus Offset 1/10 -> Multiple and Add Offset 1/19(Pixel 9)  "<signal10>"
  Pixel Bus Offset 1/8 -> Multiple and Add Offset 1/15(Pixel 7)  "<signal8>"
  Pixel Bus Offset 1/12 -> Multiple and Add Offset 1/23(Pixel 11)  "<signal12>"
  Weight Bus Offset 1/7 -> Multiple and Add Offset 1/14(Weight 6)  "<signal7>"
  Weight Bus Offset 1/2 -> Multiple and Add Offset 1/4(Weight 1)  "<signal2>"
  Pixel Bus Offset 1/9 -> Multiple and Add Offset 1/17(Pixel 8)  "<signal9>"
  Weight Bus Offset 2/5 -> Multiple and Add Offset 2/10(Weight 4)  "<signal5>"
  Pixel Bus Offset 2/7 -> Multiple and Add Offset 2/13(Pixel 6)  "<signal7>"
  Pixel Bus Offset 2/6 -> Multiple and Add Offset 2/11(Pixel 5)  "<signal6>"
  Pixel Bus Offset 2/5 -> Multiple and Add Offset 2/9(Pixel 4)  "<signal5>"
  Pixel Bus Offset 2/3 -> Multiple and Add Offset 2/5(Pixel 2)  "<signal3>"
  Pixel Bus Offset 2/11 -> Multiple and Add Offset 2/21(Pixel 10)  "<signal11>"
  Weight Bus Offset 2/6 -> Multiple and Add Offset 2/12(Weight 5)  "<signal6>"
  Pixel Bus Offset 2/2 -> Multiple and Add Offset 2/3(Pixel 1)  "<signal2>"
  Weight Bus Offset 2/12 -> Multiple and Add Offset 2/24(Weight 11)  "<signal12>"
  Weight Bus Offset 2/1 -> Multiple and Add Offset 2/2(Weight 0)  "<signal1>"
  Pixel Bus Input Offset 2/1 -> Pixel Bus Offset 2/1
  Pixel Bus Offset 2/4 -> Multiple and Add Offset 2/7(Pixel 3)  "<signal4>"
  Weight Bus Offset 2/9 -> Multiple and Add Offset 2/18(Weight 8)  "<signal9>"
  Weight Bus Offset 2/10 -> Multiple and Add Offset 2/20(Weight 9)  "<signal10>"
  Weight Bus Offset 2/11 -> Multiple and Add Offset 2/22(Weight 10)  "<signal11>"
  Weight Bus Offset 2/4 -> Multiple and Add Offset 2/8(Weight 3)  "<signal4>"
  Pixel Bus Offset 2/1 -> Multiple and Add Offset 2/1(Pixel 0)  "<signal1>"
  Weight Bus Offset 2/8 -> Multiple and Add Offset 2/16(Weight 7)  "<signal8>"
  Weight Bus Offset 2/3 -> Multiple and Add Offset 2/6(Weight 2)  "<signal3>"
  Pixel Bus Offset 2/10 -> Multiple and Add Offset 2/19(Pixel 9)  "<signal10>"
  Pixel Bus Offset 2/8 -> Multiple and Add Offset 2/15(Pixel 7)  "<signal8>"
  Pixel Bus Offset 2/12 -> Multiple and Add Offset 2/23(Pixel 11)  "<signal12>"
  Weight Bus Offset 2/7 -> Multiple and Add Offset 2/14(Weight 6)  "<signal7>"
  Weight Bus Offset 2/2 -> Multiple and Add Offset 2/4(Weight 1)  "<signal2>"
  Pixel Bus Offset 2/9 -> Multiple and Add Offset 2/17(Pixel 8)  "<signal9>"
  Weight Bus Offset 3/5 -> Multiple and Add Offset 3/10(Weight 4)  "<signal5>"
  Pixel Bus Offset 3/7 -> Multiple and Add Offset 3/13(Pixel 6)  "<signal7>"
  Pixel Bus Offset 3/6 -> Multiple and Add Offset 3/11(Pixel 5)  "<signal6>"
  Pixel Bus Offset 3/5 -> Multiple and Add Offset 3/9(Pixel 4)  "<signal5>"
  Pixel Bus Offset 3/3 -> Multiple and Add Offset 3/5(Pixel 2)  "<signal3>"
  Pixel Bus Offset 3/11 -> Multiple and Add Offset 3/21(Pixel 10)  "<signal11>"
  Weight Bus Offset 3/6 -> Multiple and Add Offset 3/12(Weight 5)  "<signal6>"
  Pixel Bus Offset 3/2 -> Multiple and Add Offset 3/3(Pixel 1)  "<signal2>"
  Weight Bus Offset 3/12 -> Multiple and Add Offset 3/24(Weight 11)  "<signal12>"
  Weight Bus Offset 3/1 -> Multiple and Add Offset 3/2(Weight 0)  "<signal1>"
  Pixel Bus Input Offset 3/1 -> Pixel Bus Offset 3/1
  Pixel Bus Offset 3/4 -> Multiple and Add Offset 3/7(Pixel 3)  "<signal4>"
  Weight Bus Offset 3/9 -> Multiple and Add Offset 3/18(Weight 8)  "<signal9>"
  Weight Bus Offset 3/10 -> Multiple and Add Offset 3/20(Weight 9)  "<signal10>"
  Weight Bus Offset 3/11 -> Multiple and Add Offset 3/22(Weight 10)  "<signal11>"
  Weight Bus Offset 3/4 -> Multiple and Add Offset 3/8(Weight 3)  "<signal4>"
  Pixel Bus Offset 3/1 -> Multiple and Add Offset 3/1(Pixel 0)  "<signal1>"
  Weight Bus Offset 3/8 -> Multiple and Add Offset 3/16(Weight 7)  "<signal8>"
  Weight Bus Offset 3/3 -> Multiple and Add Offset 3/6(Weight 2)  "<signal3>"
  Pixel Bus Offset 3/10 -> Multiple and Add Offset 3/19(Pixel 9)  "<signal10>"
  Pixel Bus Offset 3/8 -> Multiple and Add Offset 3/15(Pixel 7)  "<signal8>"
  Pixel Bus Offset 3/12 -> Multiple and Add Offset 3/23(Pixel 11)  "<signal12>"
  Weight Bus Offset 3/7 -> Multiple and Add Offset 3/14(Weight 6)  "<signal7>"
  Weight Bus Offset 3/2 -> Multiple and Add Offset 3/4(Weight 1)  "<signal2>"
  Pixel Bus Offset 3/9 -> Multiple and Add Offset 3/17(Pixel 8)  "<signal9>"
  Weight Bus Offset 4/5 -> Multiple and Add Offset 4/10(Weight 4)  "<signal5>"
  Pixel Bus Offset 4/7 -> Multiple and Add Offset 4/13(Pixel 6)  "<signal7>"
  Pixel Bus Offset 4/6 -> Multiple and Add Offset 4/11(Pixel 5)  "<signal6>"
  Pixel Bus Offset 4/5 -> Multiple and Add Offset 4/9(Pixel 4)  "<signal5>"
  Pixel Bus Offset 4/3 -> Multiple and Add Offset 4/5(Pixel 2)  "<signal3>"
  Pixel Bus Offset 4/11 -> Multiple and Add Offset 4/21(Pixel 10)  "<signal11>"
  Weight Bus Offset 4/6 -> Multiple and Add Offset 4/12(Weight 5)  "<signal6>"
  Pixel Bus Offset 4/2 -> Multiple and Add Offset 4/3(Pixel 1)  "<signal2>"
  Weight Bus Offset 4/12 -> Multiple and Add Offset 4/24(Weight 11)  "<signal12>"
  Weight Bus Offset 4/1 -> Multiple and Add Offset 4/2(Weight 0)  "<signal1>"
  Pixel Bus Input Offset 4/1 -> Pixel Bus Offset 4/1
  Pixel Bus Offset 4/4 -> Multiple and Add Offset 4/7(Pixel 3)  "<signal4>"
  Weight Bus Offset 4/9 -> Multiple and Add Offset 4/18(Weight 8)  "<signal9>"
  Weight Bus Offset 4/10 -> Multiple and Add Offset 4/20(Weight 9)  "<signal10>"
  Weight Bus Offset 4/11 -> Multiple and Add Offset 4/22(Weight 10)  "<signal11>"
  Weight Bus Offset 4/4 -> Multiple and Add Offset 4/8(Weight 3)  "<signal4>"
  Pixel Bus Offset 4/1 -> Multiple and Add Offset 4/1(Pixel 0)  "<signal1>"
  Weight Bus Offset 4/8 -> Multiple and Add Offset 4/16(Weight 7)  "<signal8>"
  Weight Bus Offset 4/3 -> Multiple and Add Offset 4/6(Weight 2)  "<signal3>"
  Pixel Bus Offset 4/10 -> Multiple and Add Offset 4/19(Pixel 9)  "<signal10>"
  Pixel Bus Offset 4/8 -> Multiple and Add Offset 4/15(Pixel 7)  "<signal8>"
  Pixel Bus Offset 4/12 -> Multiple and Add Offset 4/23(Pixel 11)  "<signal12>"
  Weight Bus Offset 4/7 -> Multiple and Add Offset 4/14(Weight 6)  "<signal7>"
  Weight Bus Offset 4/2 -> Multiple and Add Offset 4/4(Weight 1)  "<signal2>"
  Pixel Bus Offset 4/9 -> Multiple and Add Offset 4/17(Pixel 8)  "<signal9>"
  Valid Bus Input/1 -> Valid Selector/1
  Valid Selector/1 -> Multiple and Add Offset 0/25(Valid Data)  "<signal1>"
  Valid Selector/2 -> Multiple and Add Offset 1/25(Valid Data)  "<signal2>"
  Valid Selector/3 -> Multiple and Add Offset 2/25(Valid Data)  "<signal3>"
  Valid Selector/4 -> Multiple and Add Offset 3/25(Valid Data)  "<signal4>"
  Valid Selector/5 -> Multiple and Add Offset 4/25(Valid Data)  "<signal5>"
  Weight Bus Input/1 -> Bus Selector/1
  Bus Selector/5 -> Weight Bus Offset 4/1  "<signal5>"
  Bus Selector/4 -> Weight Bus Offset 3/1  "<signal4>"
  Bus Selector/3 -> Weight Bus Offset 2/1  "<signal3>"
  Bus Selector/2 -> Weight Bus Offset 1/1  "<signal2>"
  Bus Selector/1 -> Weight Bus Offset 0/1  "<signal1>"
  Delay Addition4/1 -> Accumulator Offset 4/3(Last Row), Accumulator Offset 3/3(Last Row), Accumulator Offset 2/3(Last Row), Accumulator Offset 1/3(Last Row), Accumulator Offset 0/3(Last Row)
  Delay Addition 2/1 -> Delay Addition2/1
  Delay Addition1/1 -> Delay Addition 2/1
  Delay Addition2/1 -> Delay Addition3/1
  Delay Addition3/1 -> Delay Addition4/1
  Bus Selector/6 -> Delay Addition1/1  "<signal6>"
  Delay Addition7/1 -> Delay Addition8/1
  Delay Addition 1/1 -> Delay Addition6/1
  Delay Addition5/1 -> Delay Addition 1/1
  Delay Addition6/1 -> Delay Addition7/1
  Delay Addition8/1 -> Accumlator Kernel Results/11(Reset Collector), Accumulator Offset 0/4(Hard Reset), Accumulator Offset 1/4(Hard Reset), Accumulator Offset 2/4(Hard Reset), Accumulator Offset 3/4(Hard Reset), Accumulator Offset 4/4(Hard Reset)
  Hard Reset/1 -> Delay Addition5/1
